simulink model "nonlineartankfmu_control101"  (R2025a)
settings: Solver=VariableStepAuto  StartTime=0.0  StopTime=300.0  RelTol=1e-3
values from neighbouring files (symbols this model uses):
  T2value = 200    [testfmu_control101.m]
settings Model: Creator=Anthony  LastModifiedBy=Anthony Rossiter

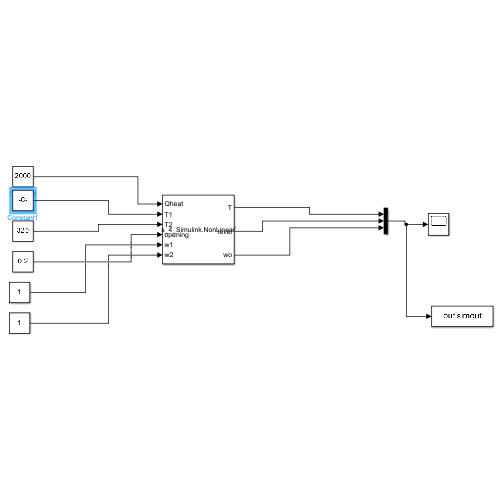
[thumbnail: Simulink's stored preview of the top-level diagram]
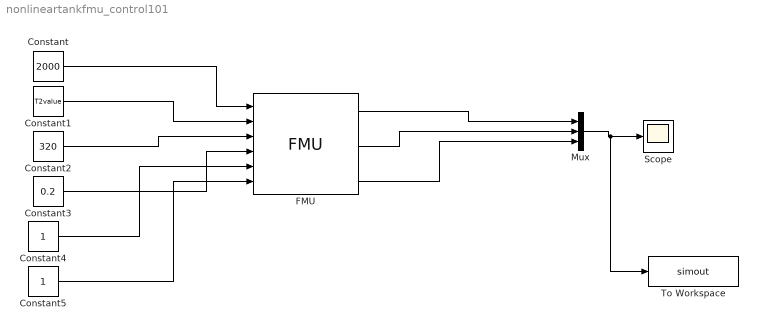
== system nonlineartankfmu_control101 ==
  Constant : Constant  Value=2000
  Constant1 : Constant  Value=T2value
  Constant2 : Constant  Value=320
  Constant3 : Constant  Value=0.2
  Constant4 : Constant
  Constant5 : Constant
  FMU : FMU  FMUName=NonLinearTank.fmu  FMUMode=CoSimulation  FMUInitializeEnumObject=off  BaseArea=0.02  SpecHeat=4186.0  T_start=300.0  kflow=2.0  level_start=0.4  ro=1000.0  mask(FMUs_4_Simulink.NonLinearTank [Co-Simulation, v2.0]){}
      mask Display:
      | disp('FMUs_4_Simulink.NonLinearTank');
      | port_label('output',1,'T');
      | port_label('output',2,'level');
      | port_label('output',3,'wo');
      | port_label('input',1,'Qheat');
      | port_label('input',2,'T1');
      | port_label('input',3,'T2');
      | port_label('input',4,'opening');
      | port_label('input',5,'w1');
      | port_label('input',6,'w2');
  Mux : Mux  Inputs=3
  Scope : Scope
      settings: ActiveDisplayYMinimum=-39.135187174942224  ActiveDisplayYMaximum=354.74650670261479
  To Workspace : ToWorkspace  VariableName=simout  SaveFormat=Structure With Time  SampleTime=-1
  wires:
  Constant/1 -> FMU/1
  Constant1/1 -> FMU/2
  Constant2/1 -> FMU/3
  Constant3/1 -> FMU/4
  Constant4/1 -> FMU/5
  Constant5/1 -> FMU/6
  FMU/2 -> Mux/2
  Mux/1 -> Scope/1, To Workspace/1
  FMU/3 -> Mux/3
  FMU/1 -> Mux/1
